simulink model "Position"  (R2016b)
settings: Solver=ode2  StartTime=0.0  StopTime=10.0  FixedStep=sample_time  RelTol=1e-3  EnableMultiTasking=on
InitFcn:
  | Parameters_quadrotor
  | Parameters_controllers
undefined symbols (not defined in the file): ALT_N, KB_D, KB_E, KB_N, KB_U, KB_V, KD_D, KD_E, KD_N, KD_U, KD_V, KI_D, KI_E, KI_N, KI_U, KI_V, KP_D, KP_E, KP_N, KP_U, KP_V, MAX_DELTA_THRUST, MAX_PITCH, MAX_ROLL, MAX_VEL, MIN_DELTA_THRUST, MIN_PITCH, MIN_ROLL, MIN_VEL, POS_N, VEL_N
libraries: simulink x5
settings Model: Creator=pela  LastModifiedBy=Mattia
settings DataIOCC: LimitDataPoints=on  SaveFormat=Array
settings OptimizationCC: LifeSpan=inf
settings DebuggingCC: SFUnexpectedBacktrackingDiag=warning  SFNoUnconditionalDefaultTransitionDiag=warning  SFExecutionAtInitializationDiag=none
settings HardwareCC: ProdBitPerPointer=32  ProdBitPerSizeT=32  ProdBitPerPtrDiffT=32  ProdLargestAtomicInteger=Long  ProdLargestAtomicFloat=Double  ProdIntDivRoundTo=Undefined  ProdWordSize=32  ProdHWDeviceType=ARM Compatible->ARM Cortex
settings ModelReferenceCC: PropagateSignalLabelsOutOfModel=off
settings RTWCC: GenCodeOnly=on  GenerateReport=on  Toolchain=GNU gcc/g++ v4.4.x | gmake (64-bit Linux)  BuildConfiguration=Faster Runs  LaunchReport=on  TargetLang=C++
settings GRTTargetCC: TargetLangStandard=C89/C90 (ANSI)  GeneratePreprocessorConditionals=Disable all  MatFileLogging=off  MultiInstanceERTCode=on  CodeInterfacePackaging=C++ class  SupportNonFinite=off
settings ConfigComp: CovMetricSettings=dw  CovHtmlReporting=on  CovSaveCumulativeToWorkspaceVar=on  CovSaveSingleToWorkspaceVar=on  CovExternalEMLEnable=off

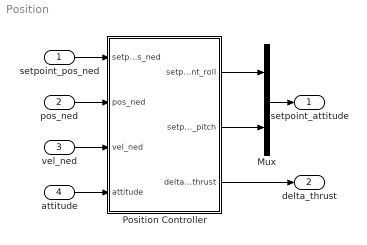
== system Position ==
  setpoint_pos_ned : Inport  PortDimensions=3
  pos_ned : Inport  Port=2  PortDimensions=3
  vel_ned : Inport  Port=3  PortDimensions=3
  attitude : Inport  Port=4
  Mux : Mux  Inputs=2
  Position Controller : Subsystem
  setpoint_attitude : Outport  PortDimensions=2
  delta_thrust : Outport  Port=2  PortDimensions=1
  wires:
  Position Controller/2(setpoint_pitch) -> Mux/2
  setpoint_pos_ned/1 -> Position Controller/1(setpoint_pos_ned)
  Position Controller/1(setpoint_roll) -> Mux/1
  attitude/1 -> Position Controller/4(attitude)
  vel_ned/1 -> Position Controller/3(vel_ned)
  pos_ned/1 -> Position Controller/2(pos_ned)
  Position Controller/3(delta_thrust) -> delta_thrust/1
  Mux/1 -> setpoint_attitude/1

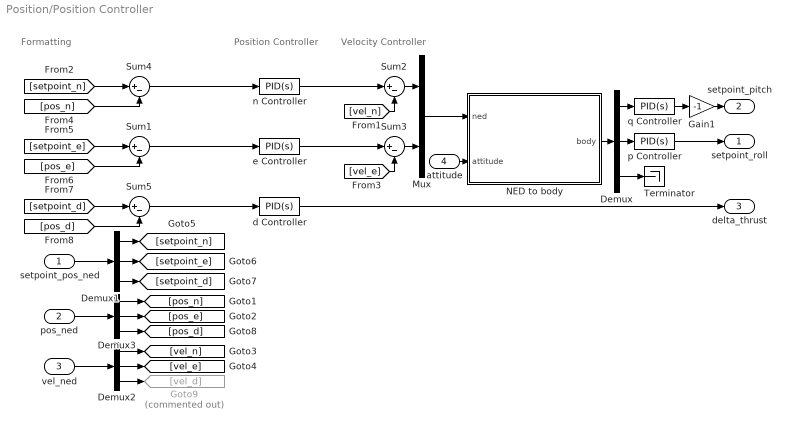
== system Position/Position Controller ==
  note: Formatting
  note: Velocity Controller
  note: Position Controller
  setpoint_pos_ned : Inport  PortDimensions=3
  pos_ned : Inport  Port=2  PortDimensions=3
  vel_ned : Inport  Port=3
  attitude : Inport  Port=4  PortDimensions=3
  Demux{,1..3} (4 alike) : Demux  Outputs=3
  Gain1 : Gain  Gain=-1
  Goto9 : Goto  Commented=on  GotoTag=vel_d
  Mux : Mux  Inputs=2
  NED to body : MATLAB Function  TreatAsAtomicUnit=on
  Sum{1..5} (5 alike) : Sum  Inputs=|+-
  Terminator : Terminator
  d Controller : simulink/Continuous/PID Controller  Controller=PID  TimeDomain=Continuous-time  SampleTime=-1  IntegratorMethod=Forward Euler  FilterMethod=Trapezoidal  Form=Parallel  UseFilter=on  ControllerParametersSource=internal  P=KP_D  I=KI_D  D=KD_D  N=ALT_N  InitialConditionSource=internal  InitialConditionForIntegrator=0  InitialConditionForFilter=0  ExternalReset=none  LimitOutput=on  UpperSaturationLimit=MAX_DELTA_THRUST  LowerSaturationLimit=MIN_DELTA_THRUST  LinearizeAsGain=on  AntiWindupMode=back-calculation  Kb=KB_D  TrackingMode=off  Kt=1  PParamMin=[]  PParamMax=[]  IParamMin=[]  IParamMax=[]  DParamMin=[]  DParamMax=[]  NParamMin=[]  NParamMax=[]  KbParamMin=[]  KbParamMax=[]  KtParamMin=[]  KtParamMax=[]  POutMin=[]  POutMax=[]  IOutMin=[]  IOutMax=[]  DOutMin=[]  DOutMax=[]  NOutMin=[]  NOutMax=[]  KbOutMin=[]  KbOutMax=[]  KtOutMin=[]  KtOutMax=[]  IntegratorOutMin=[]  IntegratorOutMax=[]  FilterOutMin=[]  FilterOutMax=[]  SumOutMin=[]  SumOutMax=[]  SumI1OutMin=[]  SumI1OutMax=[]  SumI2OutMin=[]  SumI2OutMax=[]  SumI3OutMin=[]  SumI3OutMax=[]  SumDOutMin=[]  SumDOutMax=[]  SaturationOutMin=[]  SaturationOutMax=[]  IntegratorContinuousStateAttributes=''  IntegratorStateMustResolveToSignalObject=off  IntegratorRTWStateStorageClass=Auto  FilterContinuousStateAttributes=''  FilterStateMustResolveToSignalObject=off  FilterRTWStateStorageClass=Auto  DifferentiatorICPrevScaledInput=0  DifferentiatorOutMin=[]  DifferentiatorOutMax=[]
  e Controller : simulink/Continuous/PID Controller  Controller=PID  TimeDomain=Continuous-time  SampleTime=-1  IntegratorMethod=Forward Euler  FilterMethod=Trapezoidal  Form=Parallel  UseFilter=on  ControllerParametersSource=internal  P=KP_E  I=KI_E  D=KD_E  N=POS_N  InitialConditionSource=internal  InitialConditionForIntegrator=0  InitialConditionForFilter=0  ExternalReset=none  LimitOutput=on  UpperSaturationLimit=MAX_VEL  LowerSaturationLimit=MIN_VEL  LinearizeAsGain=on  AntiWindupMode=back-calculation  Kb=KB_E  TrackingMode=off  Kt=1  PParamMin=[]  PParamMax=[]  IParamMin=[]  IParamMax=[]  DParamMin=[]  DParamMax=[]  NParamMin=[]  NParamMax=[]  KbParamMin=[]  KbParamMax=[]  KtParamMin=[]  KtParamMax=[]  POutMin=[]  POutMax=[]  IOutMin=[]  IOutMax=[]  DOutMin=[]  DOutMax=[]  NOutMin=[]  NOutMax=[]  KbOutMin=[]  KbOutMax=[]  KtOutMin=[]  KtOutMax=[]  IntegratorOutMin=[]  IntegratorOutMax=[]  FilterOutMin=[]  FilterOutMax=[]  SumOutMin=[]  SumOutMax=[]  SumI1OutMin=[]  SumI1OutMax=[]  SumI2OutMin=[]  SumI2OutMax=[]  SumI3OutMin=[]  SumI3OutMax=[]  SumDOutMin=[]  SumDOutMax=[]  SaturationOutMin=[]  SaturationOutMax=[]  IntegratorContinuousStateAttributes=''  IntegratorStateMustResolveToSignalObject=off  IntegratorRTWStateStorageClass=Auto  FilterContinuousStateAttributes=''  FilterStateMustResolveToSignalObject=off  FilterRTWStateStorageClass=Auto  DifferentiatorICPrevScaledInput=0  DifferentiatorOutMin=[]  DifferentiatorOutMax=[]
  n Controller : simulink/Continuous/PID Controller  Controller=PID  TimeDomain=Continuous-time  SampleTime=-1  IntegratorMethod=Forward Euler  FilterMethod=Trapezoidal  Form=Parallel  UseFilter=on  ControllerParametersSource=internal  P=KP_N  I=KI_N  D=KD_N  N=POS_N  InitialConditionSource=internal  InitialConditionForIntegrator=0  InitialConditionForFilter=0  ExternalReset=none  LimitOutput=on  UpperSaturationLimit=MAX_VEL  LowerSaturationLimit=MIN_VEL  LinearizeAsGain=on  AntiWindupMode=back-calculation  Kb=KB_N  TrackingMode=off  Kt=1  PParamMin=[]  PParamMax=[]  IParamMin=[]  IParamMax=[]  DParamMin=[]  DParamMax=[]  NParamMin=[]  NParamMax=[]  KbParamMin=[]  KbParamMax=[]  KtParamMin=[]  KtParamMax=[]  POutMin=[]  POutMax=[]  IOutMin=[]  IOutMax=[]  DOutMin=[]  DOutMax=[]  NOutMin=[]  NOutMax=[]  KbOutMin=[]  KbOutMax=[]  KtOutMin=[]  KtOutMax=[]  IntegratorOutMin=[]  IntegratorOutMax=[]  FilterOutMin=[]  FilterOutMax=[]  SumOutMin=[]  SumOutMax=[]  SumI1OutMin=[]  SumI1OutMax=[]  SumI2OutMin=[]  SumI2OutMax=[]  SumI3OutMin=[]  SumI3OutMax=[]  SumDOutMin=[]  SumDOutMax=[]  SaturationOutMin=[]  SaturationOutMax=[]  IntegratorContinuousStateAttributes=''  IntegratorStateMustResolveToSignalObject=off  IntegratorRTWStateStorageClass=Auto  FilterContinuousStateAttributes=''  FilterStateMustResolveToSignalObject=off  FilterRTWStateStorageClass=Auto  DifferentiatorICPrevScaledInput=0  DifferentiatorOutMin=[]  DifferentiatorOutMax=[]
  p Controller : simulink/Continuous/PID Controller  Controller=PID  TimeDomain=Continuous-time  SampleTime=-1  IntegratorMethod=Forward Euler  FilterMethod=Trapezoidal  Form=Parallel  UseFilter=on  ControllerParametersSource=internal  P=KP_V  I=KI_V  D=KD_V  N=VEL_N  InitialConditionSource=internal  InitialConditionForIntegrator=0  InitialConditionForFilter=0  ExternalReset=none  LimitOutput=on  UpperSaturationLimit=MAX_ROLL  LowerSaturationLimit=MIN_ROLL  LinearizeAsGain=on  AntiWindupMode=back-calculation  Kb=KB_V  TrackingMode=off  Kt=1  PParamMin=[]  PParamMax=[]  IParamMin=[]  IParamMax=[]  DParamMin=[]  DParamMax=[]  NParamMin=[]  NParamMax=[]  KbParamMin=[]  KbParamMax=[]  KtParamMin=[]  KtParamMax=[]  POutMin=[]  POutMax=[]  IOutMin=[]  IOutMax=[]  DOutMin=[]  DOutMax=[]  NOutMin=[]  NOutMax=[]  KbOutMin=[]  KbOutMax=[]  KtOutMin=[]  KtOutMax=[]  IntegratorOutMin=[]  IntegratorOutMax=[]  FilterOutMin=[]  FilterOutMax=[]  SumOutMin=[]  SumOutMax=[]  SumI1OutMin=[]  SumI1OutMax=[]  SumI2OutMin=[]  SumI2OutMax=[]  SumI3OutMin=[]  SumI3OutMax=[]  SumDOutMin=[]  SumDOutMax=[]  SaturationOutMin=[]  SaturationOutMax=[]  IntegratorContinuousStateAttributes=''  IntegratorStateMustResolveToSignalObject=off  IntegratorRTWStateStorageClass=Auto  FilterContinuousStateAttributes=''  FilterStateMustResolveToSignalObject=off  FilterRTWStateStorageClass=Auto  DifferentiatorICPrevScaledInput=0  DifferentiatorOutMin=[]  DifferentiatorOutMax=[]
  q Controller : simulink/Continuous/PID Controller  Controller=PID  TimeDomain=Continuous-time  SampleTime=-1  IntegratorMethod=Forward Euler  FilterMethod=Trapezoidal  Form=Parallel  UseFilter=on  ControllerParametersSource=internal  P=KP_U  I=KI_U  D=KD_U  N=VEL_N  InitialConditionSource=internal  InitialConditionForIntegrator=0  InitialConditionForFilter=0  ExternalReset=none  LimitOutput=on  UpperSaturationLimit=MAX_PITCH  LowerSaturationLimit=MIN_PITCH  LinearizeAsGain=on  AntiWindupMode=back-calculation  Kb=KB_U  TrackingMode=off  Kt=1  PParamMin=[]  PParamMax=[]  IParamMin=[]  IParamMax=[]  DParamMin=[]  DParamMax=[]  NParamMin=[]  NParamMax=[]  KbParamMin=[]  KbParamMax=[]  KtParamMin=[]  KtParamMax=[]  POutMin=[]  POutMax=[]  IOutMin=[]  IOutMax=[]  DOutMin=[]  DOutMax=[]  NOutMin=[]  NOutMax=[]  KbOutMin=[]  KbOutMax=[]  KtOutMin=[]  KtOutMax=[]  IntegratorOutMin=[]  IntegratorOutMax=[]  FilterOutMin=[]  FilterOutMax=[]  SumOutMin=[]  SumOutMax=[]  SumI1OutMin=[]  SumI1OutMax=[]  SumI2OutMin=[]  SumI2OutMax=[]  SumI3OutMin=[]  SumI3OutMax=[]  SumDOutMin=[]  SumDOutMax=[]  SaturationOutMin=[]  SaturationOutMax=[]  IntegratorContinuousStateAttributes=''  IntegratorStateMustResolveToSignalObject=off  IntegratorRTWStateStorageClass=Auto  FilterContinuousStateAttributes=''  FilterStateMustResolveToSignalObject=off  FilterRTWStateStorageClass=Auto  DifferentiatorICPrevScaledInput=0  DifferentiatorOutMin=[]  DifferentiatorOutMax=[]
  setpoint_roll : Outport  PortDimensions=1
  setpoint_pitch : Outport  Port=2  PortDimensions=1
  delta_thrust : Outport  Port=3
  wires:
  p Controller/1 -> setpoint_roll/1
  attitude/1 -> NED to body/2(attitude)
  pos_ned/1 -> Demux3/1
  Demux2/1 -> [vel_n]
  Demux2/2 -> [vel_e]
  vel_ned/1 -> Demux2/1
  q Controller/1 -> Gain1/1
  Gain1/1 -> setpoint_pitch/1
  setpoint_pos_ned/1 -> Demux1/1
  Demux3/1 -> [pos_n]
  Demux3/2 -> [pos_e]
  Demux1/1 -> [setpoint_n]
  Demux1/2 -> [setpoint_e]
  [setpoint_n] -> Sum4/1
  [pos_n] -> Sum4/2
  [setpoint_e] -> Sum1/1
  Mux/1 -> NED to body/1(ned)
  NED to body/1(body) -> Demux/1
  Demux/1 -> q Controller/1
  Demux/2 -> p Controller/1
  Sum4/1 -> n Controller/1
  Sum1/1 -> e Controller/1
  Demux/3 -> Terminator/1
  n Controller/1 -> Sum2/1
  Sum2/1 -> Mux/1
  [vel_n] -> Sum2/2
  Sum3/1 -> Mux/2
  e Controller/1 -> Sum3/1
  [vel_e] -> Sum3/2
  [pos_e] -> Sum1/2
  d Controller/1 -> delta_thrust/1
  Demux1/3 -> [setpoint_d]
  Demux3/3 -> [pos_d]
  Demux2/3 -> Goto9/1
  Sum5/1 -> d Controller/1
  [pos_d] -> Sum5/2
  [setpoint_d] -> Sum5/1

== matlab function Position/Position Controller/NED to body ==
  data: ned input; attitude input; body output
function body  = ned2body(ned,attitude)

phi = 0;
theta = 0;
psi = attitude(3);

Vel_NED = [ned(1) ;
    ned(2) ;
    0];

Sphi = sin(phi);
Cphi = cos(phi);
Stheta = sin(theta);
Ctheta = cos(theta);
Spsi = sin(psi);
Cpsi = cos(psi);

ned2body = [        Ctheta*Cpsi               Ctheta*Spsi          -Stheta;
       Sphi*Stheta*Cpsi-Cphi*Spsi Sphi*Stheta*Spsi+Cphi*Cpsi Sphi*Ctheta ;
       Cphi*Stheta*Cpsi+Sphi*Spsi Cphi*Stheta*Spsi-Sphi*Cpsi Cphi*Ctheta];

body = ned2body * Vel_NED;
